simulink model "RelayTest"  (R2018a)
settings: Solver=VariableStepAuto  StartTime=0.0  StopTime=30.0  RelTol=1e-3
undefined symbols (not defined in the file or in its folder): Gs
libraries: cstblocks x4
settings Model: Creator=xiangyuliu  LastModifiedBy=xiangyuliu

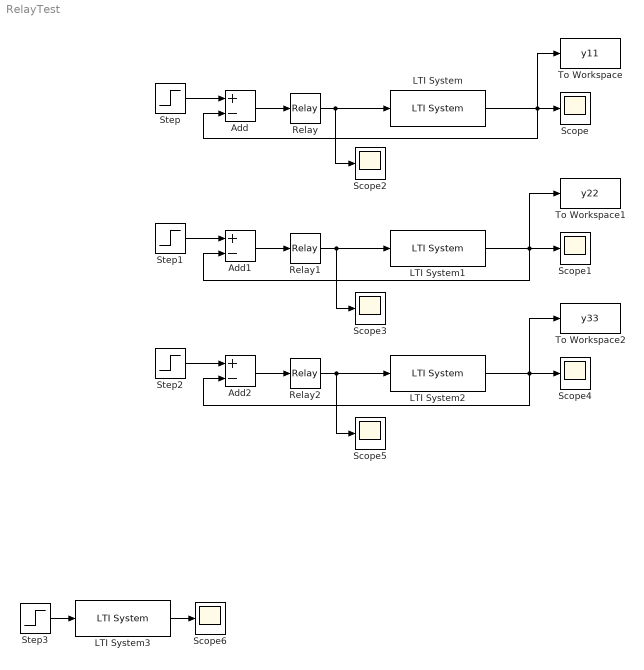
== system RelayTest ==
  Add : Sum  Inputs=+-
  Add1 : Sum  Inputs=+-
  Add2 : Sum  Inputs=+-
  LTI System : cstblocks/LTI System  sys=Gs(1,1)  IC=[]
  LTI System1 : cstblocks/LTI System  sys=Gs(3,2)  IC=[]
  LTI System2 : cstblocks/LTI System  sys=Gs(2,3)  IC=[]
  LTI System3 : cstblocks/LTI System  sys=Gs(2,2)  IC=[]
  Relay : Relay  OnSwitchValue=1  OffSwitchValue=1  OnOutputValue=-1  OffOutputValue=1
  Relay1 : Relay  OnSwitchValue=1  OffSwitchValue=1  OnOutputValue=-1  OffOutputValue=1
  Relay2 : Relay  OnSwitchValue=1  OffSwitchValue=1  OffOutputValue=-1
  Scope{,1..6} (7 alike) : Scope
  Step{,1..3} (4 alike) : Step  Time=0  SampleTime=0
  To Workspace : ToWorkspace  VariableName=y11  SaveFormat=Timeseries  SampleTime=-1
  To Workspace1 : ToWorkspace  VariableName=y22  SaveFormat=Timeseries  SampleTime=-1
  To Workspace2 : ToWorkspace  VariableName=y33  SaveFormat=Timeseries  SampleTime=-1
  wires:
  Add/1 -> Relay/1
  Step/1 -> Add/1
  Step1/1 -> Add1/1
  LTI System1/1 -> Add1/2, To Workspace1/1, Scope1/1
  Add1/1 -> Relay1/1
  Relay1/1 -> LTI System1/1, Scope3/1
  LTI System2/1 -> Add2/2, To Workspace2/1, Scope4/1
  Step2/1 -> Add2/1
  Add2/1 -> Relay2/1
  Relay2/1 -> LTI System2/1, Scope5/1
  Relay/1 -> LTI System/1, Scope2/1
  LTI System/1 -> To Workspace/1, Scope/1, Add/2
  Step3/1 -> LTI System3/1
  LTI System3/1 -> Scope6/1
